simulink model "integrated_energy_system"  (R2024b)
settings: Solver=FixedStepDiscrete  StartTime=0.0  StopTime=0.5  FixedStep=1e-4  RelTol=1e-3
settings Model: Creator=SESA504213  LastModifiedBy=SESA504213

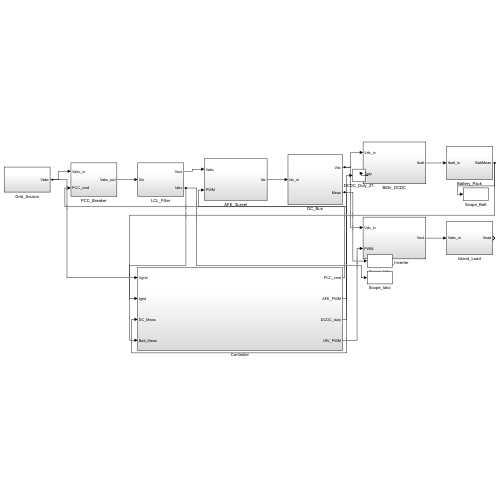
[thumbnail: Simulink's stored preview of the top-level diagram]
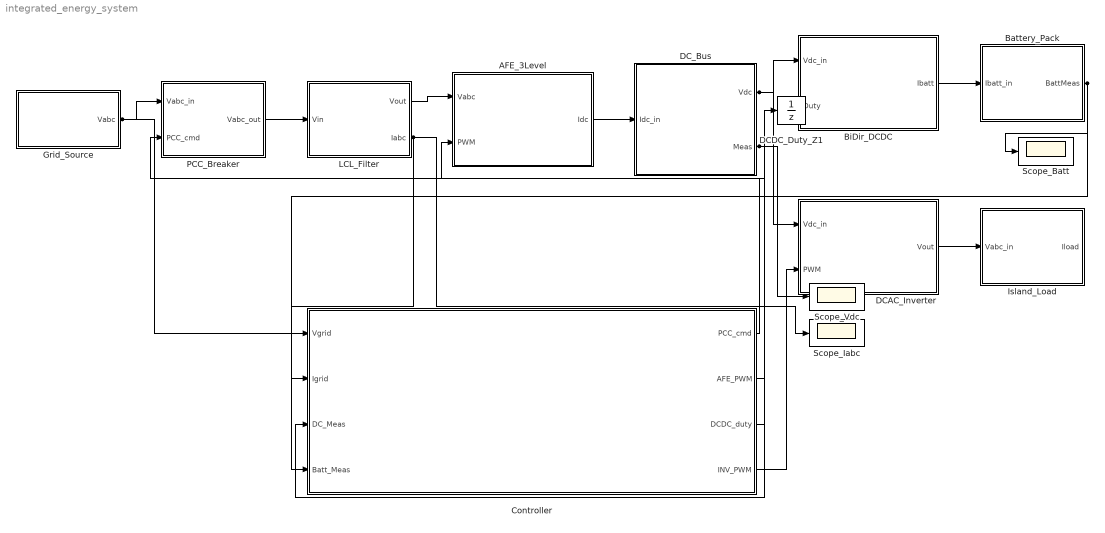
== system integrated_energy_system ==
  AFE_3Level : Subsystem
  Battery_Pack : Subsystem
  BiDir_DCDC : Subsystem
  Controller : Subsystem
  DCAC_Inverter : Subsystem
  DCDC_Duty_Z1 : UnitDelay  SampleTime=1e-4  HasFrameUpgradeWarning=on
  DC_Bus : Subsystem
  Grid_Source : Subsystem
  Island_Load : Subsystem
  LCL_Filter : Subsystem
  PCC_Breaker : Subsystem
  Scope_Batt : Scope
  Scope_Iabc : Scope
  Scope_Vdc : Scope
  wires:
  Grid_Source/1(Vabc) -> PCC_Breaker/1(Vabc_in), Controller/1(Vgrid)
  PCC_Breaker/1(Vabc_out) -> LCL_Filter/1(Vin)
  LCL_Filter/1(Vout) -> AFE_3Level/1(Vabc)
  AFE_3Level/1(Idc) -> DC_Bus/1(Idc_in)
  DC_Bus/1(Vdc) -> BiDir_DCDC/1(Vdc_in), DCAC_Inverter/1(Vdc_in)
  BiDir_DCDC/1(Ibatt) -> Battery_Pack/1(Ibatt_in)
  DCAC_Inverter/1(Vout) -> Island_Load/1(Vabc_in)
  LCL_Filter/2(Iabc) -> Controller/2(Igrid), Scope_Iabc/1
  DC_Bus/2(Meas) -> Controller/3(DC_Meas), Scope_Vdc/1
  Battery_Pack/1(BattMeas) -> Controller/4(Batt_Meas), Scope_Batt/1
  Controller/1(PCC_cmd) -> PCC_Breaker/2(PCC_cmd)
  Controller/2(AFE_PWM) -> AFE_3Level/2(PWM)
  Controller/3(DCDC_duty) -> DCDC_Duty_Z1/1
  DCDC_Duty_Z1/1 -> BiDir_DCDC/2(Duty)
  Controller/4(INV_PWM) -> DCAC_Inverter/2(PWM)

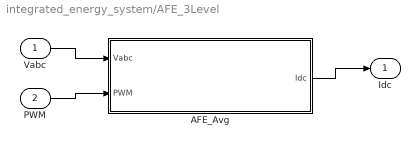
== system integrated_energy_system/AFE_3Level ==
  Vabc : Inport
  PWM : Inport  Port=2
  AFE_Avg : MATLAB Function  TreatAsAtomicUnit=on
  Idc : Outport
  wires:
  Vabc/1 -> AFE_Avg/1(Vabc)
  PWM/1 -> AFE_Avg/2(PWM)
  AFE_Avg/1(Idc) -> Idc/1

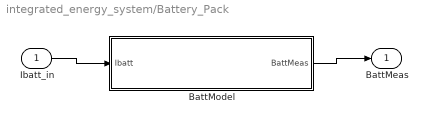
== system integrated_energy_system/Battery_Pack ==
  Ibatt_in : Inport
  BattModel : MATLAB Function  TreatAsAtomicUnit=on
  BattMeas : Outport
  wires:
  Ibatt_in/1 -> BattModel/1(Ibatt)
  BattModel/1(BattMeas) -> BattMeas/1

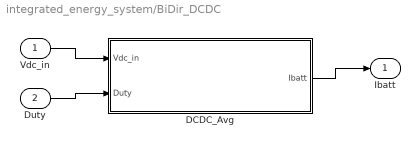
== system integrated_energy_system/BiDir_DCDC ==
  Vdc_in : Inport
  Duty : Inport  Port=2
  DCDC_Avg : MATLAB Function  TreatAsAtomicUnit=on
  Ibatt : Outport
  wires:
  Vdc_in/1 -> DCDC_Avg/1(Vdc_in)
  Duty/1 -> DCDC_Avg/2(Duty)
  DCDC_Avg/1(Ibatt) -> Ibatt/1

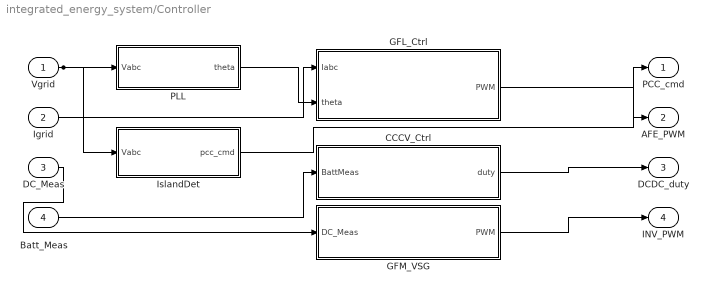
== system integrated_energy_system/Controller ==
  Vgrid : Inport
  Igrid : Inport  Port=2
  DC_Meas : Inport  Port=3
  Batt_Meas : Inport  Port=4
  CCCV_Ctrl : MATLAB Function  TreatAsAtomicUnit=on
  GFL_Ctrl : MATLAB Function  TreatAsAtomicUnit=on
  GFM_VSG : MATLAB Function  TreatAsAtomicUnit=on
  IslandDet : MATLAB Function  TreatAsAtomicUnit=on
  PLL : MATLAB Function  TreatAsAtomicUnit=on
  PCC_cmd : Outport
  AFE_PWM : Outport  Port=2
  DCDC_duty : Outport  Port=3
  INV_PWM : Outport  Port=4
  wires:
  Vgrid/1 -> PLL/1(Vabc), IslandDet/1(Vabc)
  Igrid/1 -> GFL_Ctrl/1(Iabc)
  PLL/1(theta) -> GFL_Ctrl/2(theta)
  Batt_Meas/1 -> CCCV_Ctrl/1(BattMeas)
  DC_Meas/1 -> GFM_VSG/1(DC_Meas)
  IslandDet/1(pcc_cmd) -> PCC_cmd/1
  GFL_Ctrl/1(PWM) -> AFE_PWM/1
  CCCV_Ctrl/1(duty) -> DCDC_duty/1
  GFM_VSG/1(PWM) -> INV_PWM/1

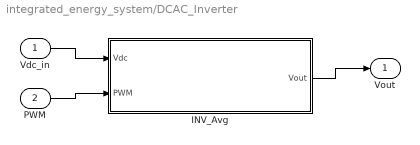
== system integrated_energy_system/DCAC_Inverter ==
  Vdc_in : Inport
  PWM : Inport  Port=2
  INV_Avg : MATLAB Function  TreatAsAtomicUnit=on
  Vout : Outport
  wires:
  Vdc_in/1 -> INV_Avg/1(Vdc)
  PWM/1 -> INV_Avg/2(PWM)
  INV_Avg/1(Vout) -> Vout/1

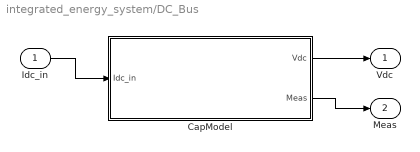
== system integrated_energy_system/DC_Bus ==
  Idc_in : Inport
  CapModel : MATLAB Function  TreatAsAtomicUnit=on
  Vdc : Outport
  Meas : Outport  Port=2
  wires:
  Idc_in/1 -> CapModel/1(Idc_in)
  CapModel/1(Vdc) -> Vdc/1
  CapModel/2(Meas) -> Meas/1

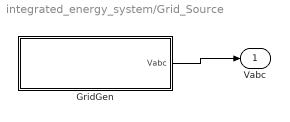
== system integrated_energy_system/Grid_Source ==
  GridGen : MATLAB Function  TreatAsAtomicUnit=on
  Vabc : Outport
  wires:
  GridGen/1(Vabc) -> Vabc/1

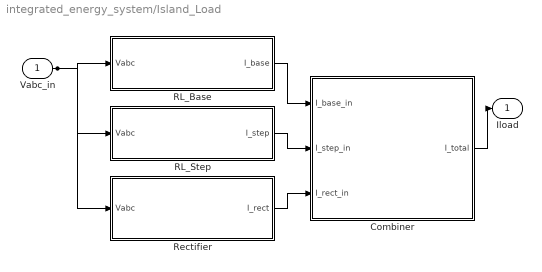
== system integrated_energy_system/Island_Load ==
  Vabc_in : Inport
  Combiner : Subsystem
  RL_Base : MATLAB Function  TreatAsAtomicUnit=on
  RL_Step : MATLAB Function  TreatAsAtomicUnit=on
  Rectifier : MATLAB Function  TreatAsAtomicUnit=on
  Iload : Outport
  wires:
  Vabc_in/1 -> RL_Base/1(Vabc), RL_Step/1(Vabc), Rectifier/1(Vabc)
  RL_Base/1(I_base) -> Combiner/1(I_base_in)
  RL_Step/1(I_step) -> Combiner/2(I_step_in)
  Rectifier/1(I_rect) -> Combiner/3(I_rect_in)
  Combiner/1(I_total) -> Iload/1

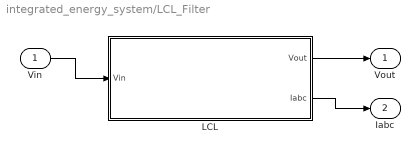
== system integrated_energy_system/LCL_Filter ==
  Vin : Inport
  LCL : MATLAB Function  TreatAsAtomicUnit=on
  Vout : Outport
  Iabc : Outport  Port=2
  wires:
  Vin/1 -> LCL/1(Vin)
  LCL/1(Vout) -> Vout/1
  LCL/2(Iabc) -> Iabc/1

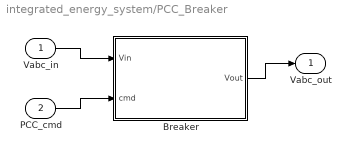
== system integrated_energy_system/PCC_Breaker ==
  Vabc_in : Inport
  PCC_cmd : Inport  Port=2
  Breaker : MATLAB Function  TreatAsAtomicUnit=on
  Vabc_out : Outport
  wires:
  Vabc_in/1 -> Breaker/1(Vin)
  PCC_cmd/1 -> Breaker/2(cmd)
  Breaker/1(Vout) -> Vabc_out/1

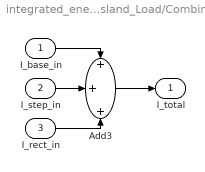
== system integrated_energy_system/Island_Load/Combiner ==
  I_base_in : Inport
  I_step_in : Inport  Port=2
  I_rect_in : Inport  Port=3
  Add3 : Sum  Inputs=+++
  I_total : Outport
  wires:
  ? -> ?
  I_base_in/1 -> Add3/1
  I_step_in/1 -> Add3/2
  I_rect_in/1 -> Add3/3
  Add3/1 -> I_total/1

== matlab function integrated_energy_system/Controller/IslandDet ==
  data: Vabc input; pcc_cmd output
function pcc_cmd = fcn(Vabc)
%#codegen
persistent tmr
if isempty(tmr), tmr = 0; end
Ts = 1e-4; Vnom = 311; V_hi = 1.1; V_lo = 0.88; t_trip = 2.0;
Vpk = max(abs(Vabc));
V_pu = Vpk / Vnom;
if V_pu > V_hi || V_pu < V_lo
    tmr = tmr + Ts;
else
    tmr = 0;
end
if tmr >= t_trip
    pcc_cmd = 0;
else
    pcc_cmd = 1;
end
end

== matlab function integrated_energy_system/Controller/CCCV_Ctrl ==
  data: BattMeas input; duty output
function duty = fcn(BattMeas)
%#codegen
persistent int_i int_v
if isempty(int_i), int_i = 0; int_v = 0; end
Ts = 1e-4; Icc = 50; Vcv = 420;
Kp_i = 0.03; Ki_i = 5; Kp_v = 1; Ki_v = 15;
Vbatt = BattMeas(1); Ibatt = BattMeas(2);
% CV loop
err_v = Vcv - Vbatt;
int_v = int_v + Ki_v*err_v*Ts;
int_v = min(max(int_v, 0), Icc);
Iref_cv = Kp_v*err_v + int_v;
Iref_cv = min(max(Iref_cv, 0), Icc);
% CC/CV min selector
Iref = min(Icc, Iref_cv);
% Current loop
err_i = Iref - Ibatt;
int_i = int_i + Ki_i*err_i*Ts;
int_i = min(max(int_i, 0), 0.95);
duty = Kp_i*err_i + int_i;
duty = min(max(duty, 0), 0.95);
end

== matlab function integrated_energy_system/Controller/GFM_VSG ==
  data: DC_Meas input; PWM output
function PWM = fcn(DC_Meas)
%#codegen
persistent th w_vsg
if isempty(th), th = 0; w_vsg = 2*pi*50; end
Ts = 1e-4; J = 0.5; D = 50; w0 = 2*pi*50; E = 311;
Vdc = DC_Meas(1);
if Vdc < 1, Vdc = 750; end
Pref = 0; Pmeas = 0;
Tm = Pref/w0; Te = Pmeas/max(w_vsg,1);
dw = (Tm - Te - D*(w_vsg-w0))/J;
w_vsg = w_vsg + dw*Ts;
w_vsg = min(max(w_vsg, 2*pi*48), 2*pi*52);
th = mod(th + w_vsg*Ts, 2*pi);
va = E*cos(th); vb = E*cos(th-2*pi/3); vc = E*cos(th+2*pi/3);
da = 0.5+va/Vdc; db = 0.5+vb/Vdc; dc = 0.5+vc/Vdc;
PWM = [min(max(da,0.05),0.95);
       min(max(db,0.05),0.95);
       min(max(dc,0.05),0.95)];
end

== matlab function integrated_energy_system/Grid_Source/GridGen ==
  data: Vabc output
function Vabc = fcn()
%#codegen
persistent t
if isempty(t), t = 0; end
Ts = 1e-4; f = 50; Vm = 311;
w = 2*pi*f;
va = Vm*cos(w*t);
vb = Vm*cos(w*t - 2*pi/3);
vc = Vm*cos(w*t + 2*pi/3);
Vabc = [va; vb; vc];
t = t + Ts;
end

== matlab function integrated_energy_system/LCL_Filter/LCL ==
  data: Vin input; Vout output; Iabc output
function [Vout, Iabc] = fcn(Vin)
%#codegen
persistent iL vC
if isempty(iL), iL = zeros(3,1); vC = zeros(3,1); end
Ts = 1e-4; L1 = 3e-3; R1 = 0.1; Cf = 10e-6;
diL = (Vin - R1*iL - vC) / L1;
iL = iL + diL * Ts;
dvC = iL / Cf;
vC = vC + dvC * Ts;
Vout = vC;
Iabc = iL;
end

== matlab function integrated_energy_system/AFE_3Level/AFE_Avg ==
  data: Vabc input; Idc output; PWM input
function Idc = fcn(Vabc, PWM)
%#codegen
% Average-value model of 3-phase PWM rectifier
% Idc = sum(duty_k * i_k), i_k from grid voltage / Zeq
persistent iL
if isempty(iL), iL = zeros(3,1); end
Ts = 1e-4; Lac = 5e-3; Rac = 0.1; Vdc_est = 750;
D = min(max(PWM, 0.05), 0.95);
Vconv = (D - 0.5) * Vdc_est;
diL = (Vabc - Vconv - Rac*iL) / Lac;
iL = iL + diL * Ts;
Idc = sum(D .* iL);
end

== matlab function integrated_energy_system/DC_Bus/CapModel ==
  data: Idc_in input; Vdc output; Meas output
function [Vdc, Meas] = fcn(Idc_in)
%#codegen
persistent vc1 vc2
if isempty(vc1), vc1 = 375; vc2 = 375; end
Ts = 1e-4; C1 = 4700e-6; C2 = 4700e-6;
% Split bus capacitor with midpoint
vc1 = vc1 + (Idc_in * 0.5) * Ts / C1;
vc2 = vc2 + (Idc_in * 0.5) * Ts / C2;
Vdc = vc1 + vc2;
Meas = [Vdc; vc1; vc2];
end

== matlab function integrated_energy_system/BiDir_DCDC/DCDC_Avg ==
  data: Vdc_in input; Ibatt output; Duty input
function Ibatt = fcn(Vdc_in, Duty)
%#codegen
persistent iL
if isempty(iL), iL = 0; end
Ts = 1e-4; L = 1e-3; R = 0.01; Vbatt_nom = 360;
D = min(max(Duty, 0), 0.95);
diL = (D * Vdc_in - Vbatt_nom - R*iL) / L;
iL = iL + diL * Ts;
iL = min(max(iL, -80), 80);
Ibatt = iL;
end

== matlab function integrated_energy_system/Battery_Pack/BattModel ==
  data: Ibatt input; BattMeas output
function BattMeas = fcn(Ibatt)
%#codegen
persistent soc
if isempty(soc), soc = 0.3; end
Ts = 1e-4; CapAh = 100; Ncells = 100; Rint = 0.001;
soc = soc + Ibatt * Ts / (CapAh * 3600);
soc = min(max(soc, 0), 1);
Voc_cell = 3.0 + 1.2*soc;
Vbatt = Ncells * (Voc_cell + Ibatt * Rint);
BattMeas = [Vbatt; Ibatt; soc];
end

== matlab function integrated_energy_system/DCAC_Inverter/INV_Avg ==
  data: Vdc input; Vout output; PWM input
function Vout = fcn(Vdc, PWM)
%#codegen
% Averaged inverter: Vout = (duty - 0.5) * Vdc
D = min(max(PWM, 0.05), 0.95);
Vout = (D - 0.5) * Vdc;
end

== matlab function integrated_energy_system/Island_Load/RL_Base ==
  data: Vabc input; I_base output
function I_base = fcn(Vabc)
%#codegen
persistent iL
if isempty(iL), iL = zeros(3,1); end
Ts = 1e-4; R = 10; L = 5e-3;
diL = (Vabc - R*iL) / L;
iL = iL + diL * Ts;
I_base = iL;
end

== matlab function integrated_energy_system/Island_Load/RL_Step ==
  data: Vabc input; I_step output
function I_step = fcn(Vabc)
%#codegen
persistent iL t_elapsed
if isempty(iL), iL = zeros(3,1); t_elapsed = 0; end
Ts = 1e-4; R_step = 15; L_step = 3e-3;
t_elapsed = t_elapsed + Ts;
% Step in at t=0.15s, magnitude = 0.5 x Ibase
if t_elapsed >= 0.15
    diL = (Vabc - R_step*iL) / L_step;
    iL = iL + diL * Ts;
else
    iL = zeros(3,1);
end
I_step = iL;
end

== matlab function integrated_energy_system/PCC_Breaker/Breaker ==
  data: Vin input; Vout output; cmd input
function Vout = fcn(Vin, cmd)
%#codegen
% PCC breaker: passes voltage when cmd >= 0.5
if cmd >= 0.5
    Vout = Vin;
else
    Vout = zeros(size(Vin));
end
end

== matlab function integrated_energy_system/Island_Load/Rectifier ==
  data: Vabc input; I_rect output
function I_rect = fcn(Vabc)
%#codegen
persistent iL3 vdc_cap
if isempty(iL3), iL3 = zeros(3,1); vdc_cap = 450; end
Ts = 1e-4; L_in = 2e-3; R_in = 0.5; C_dc = 1000e-6; R_load = 20;
Vf = 0.7; Vdc_thresh = 400;
%% AC-side inductor (simplified rectifier input)
for k = 1:3
    diL = (Vabc(k) - R_in*iL3(k)) / L_in;
    iL3(k) = iL3(k) + diL * Ts;
    % Diode clipping: only conduct when AC > DC
    if abs(Vabc(k)) < (vdc_cap - Vf)
        iL3(k) = max(iL3(k), 0);
    end
end
%% DC-side capacitor model
I_dc_avg = mean(abs(iL3));
dvdc = (I_dc_avg - vdc_cap/R_load) * Ts / C_dc;
vdc_cap = vdc_cap + dvdc;
vdc_cap = min(max(vdc_cap, 300), 650);
I_rect = iL3;
end

== matlab function integrated_energy_system/Controller/PLL ==
  data: Vabc input; theta output
function theta = fcn(Vabc)
%#codegen
persistent th integ
if isempty(th), th = 0; integ = 0; end
Ts = 1e-4; Kp = 100; Ki = 5000; w0 = 2*pi*50;
va = Vabc(1); vb = Vabc(2); vc = Vabc(3);
v_alpha = 2/3*(va - 0.5*vb - 0.5*vc);
v_beta = 2/3*(sqrt(3)/2*vb - sqrt(3)/2*vc);
vq = -v_alpha*sin(th) + v_beta*cos(th);
integ = integ + Ki*vq*Ts;
w_est = Kp*vq + integ + w0;
th = th + w_est*Ts;
th = mod(th, 2*pi);
theta = th;
end

== matlab function integrated_energy_system/Controller/GFL_Ctrl ==
  data: Iabc input; PWM output; theta input
function PWM = fcn(Iabc, theta)
%#codegen
persistent int_d int_q
if isempty(int_d), int_d = 0; int_q = 0; end
Ts = 1e-4; Kp = 10; Ki = 100; Lf = 3e-3; Vdc = 750;
w = 2*pi*50;
ia = Iabc(1); ib = Iabc(2); ic = Iabc(3);
i_al = 2/3*(ia-0.5*ib-0.5*ic);
i_be = 2/3*(sqrt(3)/2*ib - sqrt(3)/2*ic);
id = i_al*cos(theta) + i_be*sin(theta);
iq = -i_al*sin(theta) + i_be*cos(theta);
id_ref = 10; iq_ref = 0;
err_d = id_ref - id; err_q = iq_ref - iq;
int_d = int_d + Ki*err_d*Ts;
int_q = int_q + Ki*err_q*Ts;
int_d = min(max(int_d,-300),300);
int_q = min(max(int_q,-300),300);
vd = Kp*err_d + int_d - w*Lf*iq;
vq = Kp*err_q + int_q + w*Lf*id;
v_al = vd*cos(theta) - vq*sin(theta);
v_be = vd*sin(theta) + vq*cos(theta);
da = 0.5 + v_al/Vdc;
db = 0.5 + (-0.5*v_al + sqrt(3)/2*v_be)/Vdc;
dc = 0.5 + (-0.5*v_al - sqrt(3)/2*v_be)/Vdc;
PWM = [min(max(da,0.05),0.95);
       min(max(db,0.05),0.95);
       min(max(dc,0.05),0.95)];
end
